simulink model "Racecar_LQR"  (R2022b)
settings: Solver=VariableStepAuto  StartTime=0.0  StopTime=10  RelTol=1e-3
values from neighbouring files (symbols this model uses):
  K = lqr(A,B,Q,R)    [Racecar_Init.m]
  x1_0 = 0    [Racecar_Init.m]
  x1_dot_0 = 0    [Racecar_Init.m]
  x2_0 = 0    [Racecar_Init.m]
  x2_dot_0 = 0    [Racecar_Init.m]
settings Model: Creator=logan  LastModifiedBy=logan

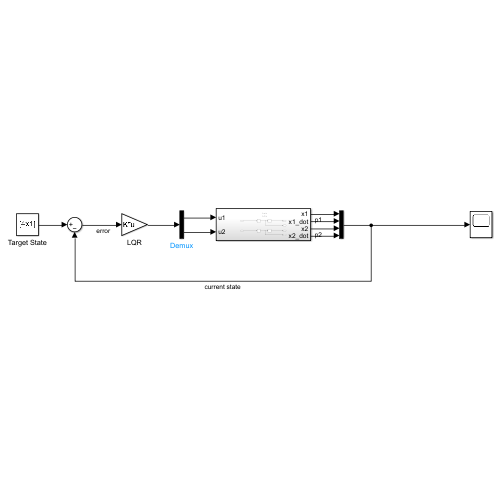
[thumbnail: Simulink's stored preview of the top-level diagram]
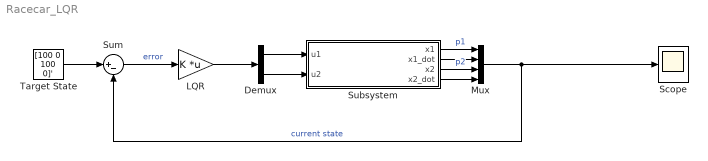
== system Racecar_LQR ==
  Demux : Demux  Outputs=2
  LQR : Gain  Gain=K  Multiplication=Matrix(K*u)
  Mux : Mux
  Scope : Scope
  Subsystem : Subsystem
  Sum : Sum  Inputs=|+-
  Target State : Constant  Value=[100 0 100 0]'
  wires:
  Target State/1 -> Sum/1
  Sum/1 -> LQR/1  "error"
  Subsystem/1(x1) -> Mux/1  "p1"
  Subsystem/2(x1_dot) -> Mux/2
  Subsystem/3(x2) -> Mux/3  "p2"
  Subsystem/4(x2_dot) -> Mux/4
  Mux/1 -> Sum/2, Scope/1  "current state"
  Demux/1 -> Subsystem/1(u1)
  Demux/2 -> Subsystem/2(u2)
  LQR/1 -> Demux/1

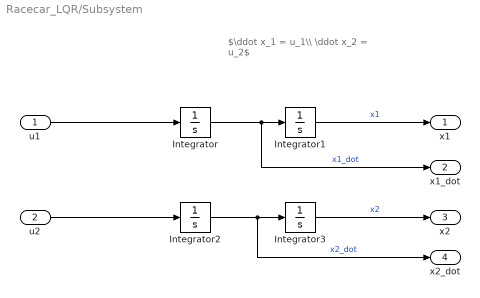
== system Racecar_LQR/Subsystem ==
  note: $\ddot x_1 = u_1\\ \ddot x_2 = u_2$
  u1 : Inport
  u2 : Inport  Port=2
  Integrator : Integrator  InitialCondition=x1_dot_0
  Integrator1 : Integrator  InitialCondition=x1_0
  Integrator2 : Integrator  InitialCondition=x2_dot_0
  Integrator3 : Integrator  InitialCondition=x2_0
  x1 : Outport
  x1_dot : Outport  Port=2
  x2 : Outport  Port=3
  x2_dot : Outport  Port=4
  wires:
  u2/1 -> Integrator2/1
  Integrator2/1 -> x2_dot/1, Integrator3/1  "x2_dot"
  Integrator3/1 -> x2/1  "x2"
  Integrator/1 -> x1_dot/1, Integrator1/1  "x1_dot"
  Integrator1/1 -> x1/1  "x1"
  u1/1 -> Integrator/1
